simulink model "pole_placement_oldversion"  (R2022a)
settings: Solver=FixedStepAuto  StartTime=0.0  StopTime=10  FixedStep=0.001  RelTol=1e-3
values from neighbouring files (symbols this model uses):
  A = [0 1.51506314161 0 -114.917471751 0 1 -372.885867158 0 797.381461885 0 0 0.563745877458 ... (25 elements, 5x5)]    [System.mat]    (also in linearize_operating_point.m = double(A))
  B = [0 0 0 0 863.333333333]    [System.mat]    (also in linearize_operating_point.m = double(B))
  C = [1  0  0  0  0; 0  0  1  0  0]    [System.mat]    (also in linearize_operating_point.m = [1 0 0 0 0)
  D = [0 0]    [System.mat]    (also in linearize_operating_point.m = zeros(2,1))
  K = K1    [controller.m]
  Ke = place(A_, B_, 2*J)'    [controller.m]
  T_0 = x_op(5)    [controller.m]    (also in run_compare_lin_non_lin.m)
  theta_1_0 = x_op(1)    [controller.m]    (also in run_compare_lin_non_lin.m)
  theta_2_0 = x_op(3)    [controller.m]    (also in run_compare_lin_non_lin.m)
  theta_d_1_0 = x_op(2)    [controller.m]    (also in run_compare_lin_non_lin.m)
  theta_d_2_0 = x_op(4)    [controller.m]    (also in run_compare_lin_non_lin.m)
  x_op = [3.14159265359 0 0 0 0]    [System.mat]    (also in linearize_operating_point.m = [init_theta_1; 0; init_theta_2; 0; 0])
  x_op_relative = [0; 0; 0; 0; 0]    [controller.m]
libraries: slpidlib x4
(part 3 of 3)

== matlab function pole_placement_oldversion/Subsystem/system_nonlinear_model2 ==
  settings: updateMethod=DISCRETE  sampleTime=0.001
  data: u input size=1; theta_dd_val output size=2; T_d output; theta_1 input size=1; theta_d_1 input size=1; theta_2 input size=1; theta_d_2 input size=1; T input; params parameter
function [theta_dd_val, T_d] = get_theta_dt_dt(u, theta_1, theta_d_1, theta_2, theta_d_2, T, params)

k_m_0 = params(7);
tau_e_0 = params(8);

T_d = -(1/tau_e_0)*T + (k_m_0/tau_e_0)*u;

% theta_dd_val = NonLinFunc(T,theta_1,theta_2,theta_d_1,theta_d_2); % this
% does not work, because simulink is stupid.

theta_dd_val = [
                                                                                                                                                                   (2177205792337185200000*sin(theta_1 + theta_2)*(7101996468378179*cos(theta_2) + 5837472162125388))/(59390441777463697512*cos(theta_2) + 157619855740175396464645510487628125*cos(theta_2)^2 - 67469767625708245300871903596602750000) - theta_d_2*((1152921504606846976*(7101996468378179*cos(theta_2) + 5837472162125388))/(59390441777463697512*cos(theta_2) + 157619855740175396464645510487628125*cos(theta_2)^2 - 67469767625708245300871903596602750000) + (336507359412909324930676272031334400000*sin(theta_2)*((7101996468378179*theta_d_1)/18446744073709551616 + (7101996468378179*theta_d_2)/18446744073709551616))/(59390441777463697512*cos(theta_2) + 157619855740175396464645510487628125*cos(theta_2)^2 - 67469767625708245300871903596602750000)) - theta_d_1*((336507359412909324930676272031334400000*((7101996468378179*theta_d_2*sin(theta_2))/18446744073709551616 - 5171/250))/(59390441777463697512*cos(theta_2) + 157619855740175396464645510487628125*cos(theta_2)^2 - 67469767625708245300871903596602750000) + (22193738963681809375*theta_d_1*sin(theta_2)*(7101996468378179*cos(theta_2) + 5837472162125388))/(59390441777463697512*cos(theta_2) + 157619855740175396464645510487628125*cos(theta_2)^2 - 67469767625708245300871903596602750000)) - (336507359412909324930676272031334400000*T)/(59390441777463697512*cos(theta_2) + 157619855740175396464645510487628125*cos(theta_2)^2 - 67469767625708245300871903596602750000) - (336507359412909324930676272031334400000*((5443014480842963*sin(theta_1 + theta_2))/144115188075855872 + (3446064362871357*sin(theta_1))/72057594037927936))/(59390441777463697512*cos(theta_2) + 157619855740175396464645510487628125*cos(theta_2)^2 - 67469767625708245300871903596602750000)
theta_d_1*((57646075230342348800000*(7101996468378179*cos(theta_2) + 5837472162125388)*((7101996468378179*theta_d_2*sin(theta_2))/18446744073709551616 - 5171/250))/(59390441777463697512*cos(theta_2) + 157619855740175396464645510487628125*cos(theta_2)^2 - 67469767625708245300871903596602750000) + (7272444383619255296*theta_d_1*sin(theta_2)*(43347146413441024*cos(theta_2) + 11304968154247740625))/(59390441777463697512*cos(theta_2) + 157619855740175396464645510487628125*cos(theta_2)^2 - 67469767625708245300871903596602750000)) + theta_d_2*((1180591620717411303424*(43347146413441024*cos(theta_2) + 11304968154247740625))/(3125*(59390441777463697512*cos(theta_2) + 157619855740175396464645510487628125*cos(theta_2)^2 - 67469767625708245300871903596602750000)) + (57646075230342348800000*sin(theta_2)*(7101996468378179*cos(theta_2) + 5837472162125388)*((7101996468378179*theta_d_1)/18446744073709551616 + (7101996468378179*theta_d_2)/18446744073709551616))/(59390441777463697512*cos(theta_2) + 157619855740175396464645510487628125*cos(theta_2)^2 - 67469767625708245300871903596602750000)) + (57646075230342348800000*T*(7101996468378179*cos(theta_2) + 5837472162125388))/(59390441777463697512*cos(theta_2) + 157619855740175396464645510487628125*cos(theta_2)^2 - 67469767625708245300871903596602750000) + (57646075230342348800000*(7101996468378179*cos(theta_2) + 5837472162125388)*((5443014480842963*sin(theta_1 + theta_2))/144115188075855872 + (3446064362871357*sin(theta_1))/72057594037927936))/(59390441777463697512*cos(theta_2) + 157619855740175396464645510487628125*cos(theta_2)^2 - 67469767625708245300871903596602750000) - (713426794033048846336*sin(theta_1 + theta_2)*(43347146413441024*cos(theta_2) + 11304968154247740625))/(59390441777463697512*cos(theta_2) + 157619855740175396464645510487628125*cos(theta_2)^2 - 67469767625708245300871903596602750000)
];

== matlab function pole_placement_oldversion/Subsystem/set_limit_rad ==
  settings: updateMethod=DISCRETE  sampleTime=0.001
  data: theta_old input size=1; theta_new output size=1
function theta_new   = set_limit_rad(theta_old)

theta_new = theta_old - floor(theta_old / 2 / pi) * 2 * pi;
theta_new = theta_old;

== matlab function pole_placement_oldversion/Subsystem/set_limit_rad1 ==
  settings: updateMethod=DISCRETE  sampleTime=0.001
  data: theta_old input size=1; theta_new output size=1
function theta_new   = set_limit_rad(theta_old)

theta_new = theta_old - floor(theta_old / 2 / pi) * 2 * pi;
theta_new = theta_old;

== matlab function pole_placement_oldversion/Subsystem/set_limit_rad2 ==
  settings: updateMethod=DISCRETE  sampleTime=0.001
  data: theta_old input size=1; theta_new output size=1
function theta_new   = set_limit_rad(theta_old)

theta_new = theta_old - floor(theta_old / 2 / pi) * 2 * pi;
theta_new = theta_old;

== matlab function pole_placement_oldversion/Subsystem/set_limit_rad3 ==
  settings: updateMethod=DISCRETE  sampleTime=0.001
  data: theta_old input size=1; theta_new output size=1
function theta_new   = set_limit_rad(theta_old)

theta_new = theta_old - floor(theta_old / 2 / pi) * 2 * pi;
theta_new = theta_old;

== matlab function pole_placement_oldversion/Subsystem/system_nonlinear_model ==
  settings: updateMethod=DISCRETE  sampleTime=0.001
  data: U input size=1; theta_dd_val output size=2; T output; theta_1 input size=1; theta_2 input size=1; theta_d_1 input size=1; theta_d_2 input size=1; T_d input; T_prev input; T_d_new output
function [theta_dd_val, T, T_d_new]   = get_theta_dt_dt(U, theta_1, theta_2, theta_d_1, theta_d_2, T_d, T_prev)


u = U(1);
k_m_0 = 15;
tau_e_0 = 0.03;

T = k_m_0 * u - tau_e_0 * T_d;



theta_dd_val = [
                                                                                                                                                                   (2177205792337185200000*sin(theta_1 + theta_2)*(7101996468378179*cos(theta_2) + 5837472162125388))/(59390441777463697512*cos(theta_2) + 157619855740175396464645510487628125*cos(theta_2)^2 - 67469767625708245300871903596602750000) - theta_d_2*((1152921504606846976*(7101996468378179*cos(theta_2) + 5837472162125388))/(59390441777463697512*cos(theta_2) + 157619855740175396464645510487628125*cos(theta_2)^2 - 67469767625708245300871903596602750000) + (336507359412909324930676272031334400000*sin(theta_2)*((7101996468378179*theta_d_1)/18446744073709551616 + (7101996468378179*theta_d_2)/18446744073709551616))/(59390441777463697512*cos(theta_2) + 157619855740175396464645510487628125*cos(theta_2)^2 - 67469767625708245300871903596602750000)) - theta_d_1*((336507359412909324930676272031334400000*((7101996468378179*theta_d_2*sin(theta_2))/18446744073709551616 - 5171/250))/(59390441777463697512*cos(theta_2) + 157619855740175396464645510487628125*cos(theta_2)^2 - 67469767625708245300871903596602750000) + (22193738963681809375*theta_d_1*sin(theta_2)*(7101996468378179*cos(theta_2) + 5837472162125388))/(59390441777463697512*cos(theta_2) + 157619855740175396464645510487628125*cos(theta_2)^2 - 67469767625708245300871903596602750000)) - (336507359412909324930676272031334400000*T)/(59390441777463697512*cos(theta_2) + 157619855740175396464645510487628125*cos(theta_2)^2 - 67469767625708245300871903596602750000) - (336507359412909324930676272031334400000*((5443014480842963*sin(theta_1 + theta_2))/144115188075855872 + (3446064362871357*sin(theta_1))/72057594037927936))/(59390441777463697512*cos(theta_2) + 157619855740175396464645510487628125*cos(theta_2)^2 - 67469767625708245300871903596602750000);
theta_d_1*((57646075230342348800000*(7101996468378179*cos(theta_2) + 5837472162125388)*((7101996468378179*theta_d_2*sin(theta_2))/18446744073709551616 - 5171/250))/(59390441777463697512*cos(theta_2) + 157619855740175396464645510487628125*cos(theta_2)^2 - 67469767625708245300871903596602750000) + (7272444383619255296*theta_d_1*sin(theta_2)*(43347146413441024*cos(theta_2) + 11304968154247740625))/(59390441777463697512*cos(theta_2) + 157619855740175396464645510487628125*cos(theta_2)^2 - 67469767625708245300871903596602750000)) + theta_d_2*((1180591620717411303424*(43347146413441024*cos(theta_2) + 11304968154247740625))/(3125*(59390441777463697512*cos(theta_2) + 157619855740175396464645510487628125*cos(theta_2)^2 - 67469767625708245300871903596602750000)) + (57646075230342348800000*sin(theta_2)*(7101996468378179*cos(theta_2) + 5837472162125388)*((7101996468378179*theta_d_1)/18446744073709551616 + (7101996468378179*theta_d_2)/18446744073709551616))/(59390441777463697512*cos(theta_2) + 157619855740175396464645510487628125*cos(theta_2)^2 - 67469767625708245300871903596602750000)) + (57646075230342348800000*T*(7101996468378179*cos(theta_2) + 5837472162125388))/(59390441777463697512*cos(theta_2) + 157619855740175396464645510487628125*cos(theta_2)^2 - 67469767625708245300871903596602750000) + (57646075230342348800000*(7101996468378179*cos(theta_2) + 5837472162125388)*((5443014480842963*sin(theta_1 + theta_2))/144115188075855872 + (3446064362871357*sin(theta_1))/72057594037927936))/(59390441777463697512*cos(theta_2) + 157619855740175396464645510487628125*cos(theta_2)^2 - 67469767625708245300871903596602750000) - (713426794033048846336*sin(theta_1 + theta_2)*(43347146413441024*cos(theta_2) + 11304968154247740625))/(59390441777463697512*cos(theta_2) + 157619855740175396464645510487628125*cos(theta_2)^2 - 67469767625708245300871903596602750000)];
 
%                                                                                                        (50632000000*((3*T_d)/100 - 15*u))/(7*(3388000*cos(theta_2)^2 - 1450246047)) - theta_d_2*((160*(7700*cos(theta_2) + 6329))/(7*(3388000*cos(theta_2)^2 - 1450246047)) + (50632000000*sin(theta_2)*((77*theta_d_1)/200000 + (77*theta_d_2)/200000))/(7*(3388000*cos(theta_2)^2 - 1450246047))) - (50632000000*((75537*sin(theta_1 + theta_2))/2000000 + (38259*sin(theta_1))/800000))/(7*(3388000*cos(theta_2)^2 - 1450246047)) - theta_d_1*((50632000000*((77*theta_d_2*sin(theta_2))/200000 - 5171/250))/(7*(3388000*cos(theta_2)^2 - 1450246047)) + (440*theta_d_1*sin(theta_2)*(7700*cos(theta_2) + 6329))/(3388000*cos(theta_2)^2 - 1450246047)) + (43164*sin(theta_1 + theta_2)*(7700*cos(theta_2) + 6329))/(3388000*cos(theta_2)^2 - 1450246047);
% theta_d_2*((80*(30800*cos(theta_2) + 8032663))/(7*(3388000*cos(theta_2)^2 - 1450246047)) + (8000000*sin(theta_2)*((77*theta_d_1)/200000 + (77*theta_d_2)/200000)*(7700*cos(theta_2) + 6329))/(7*(3388000*cos(theta_2)^2 - 1450246047))) + theta_d_1*((8000000*((77*theta_d_2*sin(theta_2))/200000 - 5171/250)*(7700*cos(theta_2) + 6329))/(7*(3388000*cos(theta_2)^2 - 1450246047)) + (220*theta_d_1*sin(theta_2)*(30800*cos(theta_2) + 8032663))/(3388000*cos(theta_2)^2 - 1450246047)) - (21582*sin(theta_1 + theta_2)*(30800*cos(theta_2) + 8032663))/(3388000*cos(theta_2)^2 - 1450246047) + (8000000*(7700*cos(theta_2) + 6329)*((75537*sin(theta_1 + theta_2))/2000000 + (38259*sin(theta_1))/800000))/(7*(3388000*cos(theta_2)^2 - 1450246047)) - (8000000*(7700*cos(theta_2) + 6329)*((3*T_d)/100 - 15*u))/(7*(3388000*cos(theta_2)^2 - 1450246047))];
%  
%                                                                                                         (43164*sin(theta_1 + theta_2)*(7700*cos(theta_2) + 6329))/(3388000*cos(theta_2)^2 - 1450246047) - (759480000000*u)/(7*(3388000*cos(theta_2)^2 - 1450246047)) - theta_d_2*((160*(7700*cos(theta_2) + 6329))/(7*(3388000*cos(theta_2)^2 - 1450246047)) + (50632000000*sin(theta_2)*((77*theta_d_1)/200000 + (77*theta_d_2)/200000))/(7*(3388000*cos(theta_2)^2 - 1450246047))) - (50632000000*((75537*sin(theta_1 + theta_2))/2000000 + (38259*sin(theta_1))/800000))/(7*(3388000*cos(theta_2)^2 - 1450246047)) - theta_d_1*((50632000000*((77*theta_d_2*sin(theta_2))/200000 - 5171/250))/(7*(3388000*cos(theta_2)^2 - 1450246047)) + (440*theta_d_1*sin(theta_2)*(7700*cos(theta_2) + 6329))/(3388000*cos(theta_2)^2 - 1450246047))
% theta_d_2*((80*(30800*cos(theta_2) + 8032663))/(7*(3388000*cos(theta_2)^2 - 1450246047)) + (8000000*sin(theta_2)*((77*theta_d_1)/200000 + (77*theta_d_2)/200000)*(7700*cos(theta_2) + 6329))/(7*(3388000*cos(theta_2)^2 - 1450246047))) + theta_d_1*((8000000*((77*theta_d_2*sin(theta_2))/200000 - 5171/250)*(7700*cos(theta_2) + 6329))/(7*(3388000*cos(theta_2)^2 - 1450246047)) + (220*theta_d_1*sin(theta_2)*(30800*cos(theta_2) + 8032663))/(3388000*cos(theta_2)^2 - 1450246047)) + (120000000*u*(7700*cos(theta_2) + 6329))/(7*(3388000*cos(theta_2)^2 - 1450246047)) - (21582*sin(theta_1 + theta_2)*(30800*cos(theta_2) + 8032663))/(3388000*cos(theta_2)^2 - 1450246047) + (8000000*(7700*cos(theta_2) + 6329)*((75537*sin(theta_1 + theta_2))/2000000 + (38259*sin(theta_1))/800000))/(7*(3388000*cos(theta_2)^2 - 1450246047))
%  

T_d_new = (T - T_prev)/1;

== matlab function pole_placement_oldversion/Subsystem1/set_limit_rad ==
  settings: updateMethod=DISCRETE  sampleTime=0.001
  data: theta_old input size=1; theta_new output size=1
function theta_new   = set_limit_rad(theta_old)

theta_new = theta_old - floor(theta_old / 2 / pi) * 2 * pi;
theta_new = theta_old;

== matlab function pole_placement_oldversion/Subsystem1/set_limit_rad1 ==
  settings: updateMethod=DISCRETE  sampleTime=0.001
  data: theta_old input size=1; theta_new output size=1
function theta_new   = set_limit_rad(theta_old)

theta_new = theta_old - floor(theta_old / 2 / pi) * 2 * pi;
theta_new = theta_old;
